simulink model "compare_filters"  (R2025a)
settings: Solver=VariableStepAuto  StartTime=0.0  StopTime=1.5  RelTol=1e-3
values from neighbouring files (symbols this model uses):
  phi_corr_LUT_param = Simulink.Parameter(phi_corr_LUT)    [lut_script.m]
undefined symbols (not defined in the file or in its folder): closed_loop, D_duty_cycle, D_m, DiscIntNeverNeededParam, hall_errors, I_duty_cycle, J_t, L_ss, lambda_m, P, P_duty_cycle, r_s, R_vs, T_m, theta_v, use_LUT, V_bus
libraries: spsMosfetLib x18, spsSeriesRLCBranchLib x12, spsVoltageMeasurementLib x9, spsControlledCurrentSourceLib x9, slpidlib x6, eeGeneralControl x3, simulink x3, embmathops x3, spsControlledVoltageSourceLib x3, spsPWMGeneratorDCDCLib x3, spsDCVoltageSourceLib x3, sps_lib x3
(part 2 of 3)

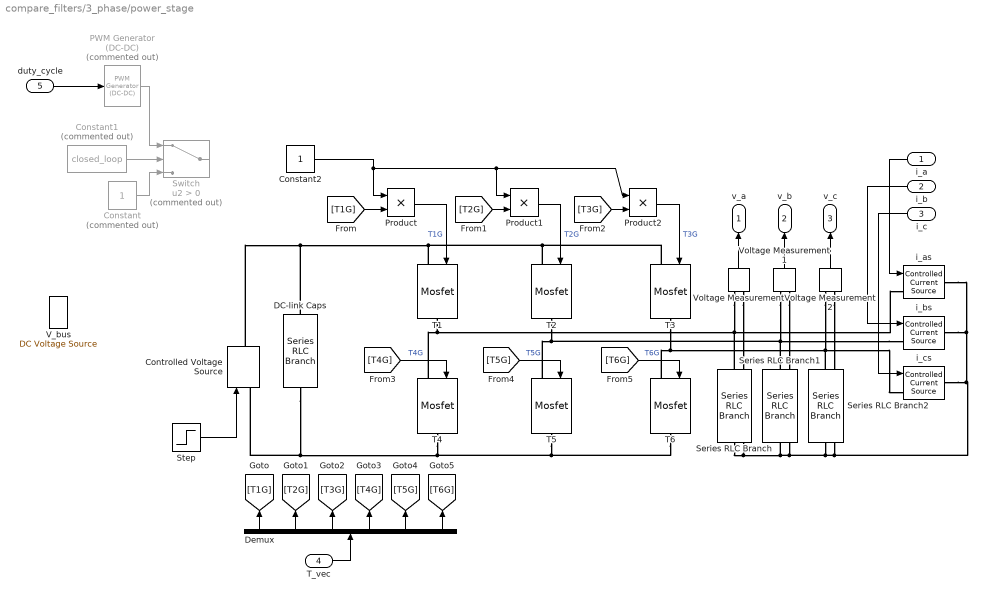
== system compare_filters/3_phase/power_stage ==
  i_a : Inport
  i_b : Inport  Port=2
  i_c : Inport  Port=3
  T_vec : Inport  Port=4
  duty_cycle : Inport  Port=5
  Constant : Constant  Commented=on
  Constant1 : Constant  Commented=on  Value=closed_loop
  Constant2 : Constant
  Controlled Voltage Source : spsControlledVoltageSourceLib/Controlled Voltage Source  Initialize=on  Source_Type=DC  Amplitude=20  Phase=0  Frequency=0  Measurements=None
  DC-link Caps : spsSeriesRLCBranchLib/Series RLC Branch  LConnTagsString=__new0  RConnTagsString=__new0  BranchType=RC  Resistance=1e-6  Inductance=0  SetiL0=off  InitialCurrent=0  Capacitance=100e-6  Setx0=off  InitialVoltage=0  Measurements=None
  Demux : Demux  Outputs=6
  PWM Generator (DC-DC) : spsPWMGeneratorDCDCLib/PWM Generator (DC-DC)  Commented=on  Fsw=f_SW_Hz  Ts=0
  Product : Product
  Product1 : Product
  Product2 : Product
  Series RLC Branch : spsSeriesRLCBranchLib/Series RLC Branch  LConnTagsString=__new0  RConnTagsString=__new0  BranchType=R  Resistance=R_vs  Inductance=0  SetiL0=off  InitialCurrent=0  Capacitance=inf  Setx0=off  InitialVoltage=0  Measurements=None
  Series RLC Branch1 : spsSeriesRLCBranchLib/Series RLC Branch  LConnTagsString=__new0  RConnTagsString=__new0  BranchType=R  Resistance=R_vs  Inductance=0  SetiL0=off  InitialCurrent=0  Capacitance=inf  Setx0=off  InitialVoltage=0  Measurements=None
  Series RLC Branch2 : spsSeriesRLCBranchLib/Series RLC Branch  LConnTagsString=__new0  RConnTagsString=__new0  BranchType=R  Resistance=R_vs  Inductance=0  SetiL0=off  InitialCurrent=0  Capacitance=inf  Setx0=off  InitialVoltage=0  Measurements=None
  Step : Step  Time=0.55  Before=20  After=35  SampleTime=0
  Switch : Switch  Commented=on  Criteria=u2 > Threshold  SaturateOnIntegerOverflow=off  InputSameDT=off
  T{1..6} (6 alike) : spsMosfetLib/Mosfet  Ron=R_dsON_Ohm  Lon=0  Rd=0.01  Vfd=0.7  IC=0  Rs=1e5  Cs=inf  Measurements=off
  V_bus : spsDCVoltageSourceLib/DC Voltage Source  Amplitude=V_bus  Measurements=None
  Voltage Measurement : spsVoltageMeasurementLib/Voltage Measurement  PhasorSimulation=off  OutputType=Complex  PSBequivalent=0
  Voltage Measurement1 : spsVoltageMeasurementLib/Voltage Measurement  PhasorSimulation=off  OutputType=Complex  PSBequivalent=0
  Voltage Measurement2 : spsVoltageMeasurementLib/Voltage Measurement  PhasorSimulation=off  OutputType=Complex  PSBequivalent=0
  i_as : spsControlledCurrentSourceLib/Controlled Current Source  Initialize=on  Source_Type=AC  Amplitude=0  Phase=0  Frequency=0  Measurements=None
  i_bs : spsControlledCurrentSourceLib/Controlled Current Source  Initialize=on  Source_Type=AC  Amplitude=0  Phase=0  Frequency=0  Measurements=None
  i_cs : spsControlledCurrentSourceLib/Controlled Current Source  Initialize=on  Source_Type=AC  Amplitude=0  Phase=0  Frequency=0  Measurements=None
  v_a : Outport
  v_b : Outport  Port=2
  v_c : Outport  Port=3
  wires:
  T_vec/1 -> Demux/1
  Product1/1 -> T2/1  "T2G"
  Constant2/1 -> Product/1, Product2/1, Product1/1
  Demux/6 -> [T6G]
  [T4G] -> T4/1  "T4G"
  [T5G] -> T5/1  "T5G"
  Demux/4 -> [T4G]
  Voltage Measurement/1 -> v_a/1
  [T2G] -> Product1/2
  Voltage Measurement1/1 -> v_b/1
  Voltage Measurement2/1 -> v_c/1
  i_a/1 -> i_as/1
  Demux/1 -> [T1G]
  Demux/5 -> [T5G]
  [T6G] -> T6/1  "T6G"
  i_c/1 -> i_cs/1
  Product/1 -> T1/1  "T1G"
  [T3G] -> Product2/2
  i_b/1 -> i_bs/1
  Product2/1 -> T3/1  "T3G"
  Demux/2 -> [T2G]
  Demux/3 -> [T3G]
  [T1G] -> Product/2
  duty_cycle/1 -> PWM Generator (DC-DC)/1
  Constant/1 -> Switch/3
  Constant1/1 -> Switch/2
  PWM Generator (DC-DC)/1 -> Switch/1
  Step/1 -> Controlled Voltage Source/1
  connections:
  i_bs/LConn1 -- Voltage Measurement1/LConn1 -- Series RLC Branch1/LConn1 -- T2/RConn1 -- T5/LConn1
  DC-link Caps/RConn1 -- Controlled Voltage Source/LConn1 -- T4/RConn1 -- T6/RConn1 -- T5/RConn1
  DC-link Caps/LConn1 -- Controlled Voltage Source/RConn1 -- T1/LConn1 -- T3/LConn1 -- T2/LConn1
  T4/LConn1 -- T1/RConn1 -- Voltage Measurement/LConn1 -- Series RLC Branch/LConn1 -- i_as/LConn1
  T3/RConn1 -- T6/LConn1 -- Voltage Measurement2/LConn1 -- Series RLC Branch2/LConn1 -- i_cs/LConn1
  Series RLC Branch/RConn1 -- Voltage Measurement/LConn2 -- i_bs/RConn1 -- i_as/RConn1 -- i_cs/RConn1 -- Voltage Measurement2/LConn2 -- Series RLC Branch2/RConn1 -- Voltage Measurement1/LConn2 -- Series RLC Branch1/RConn1

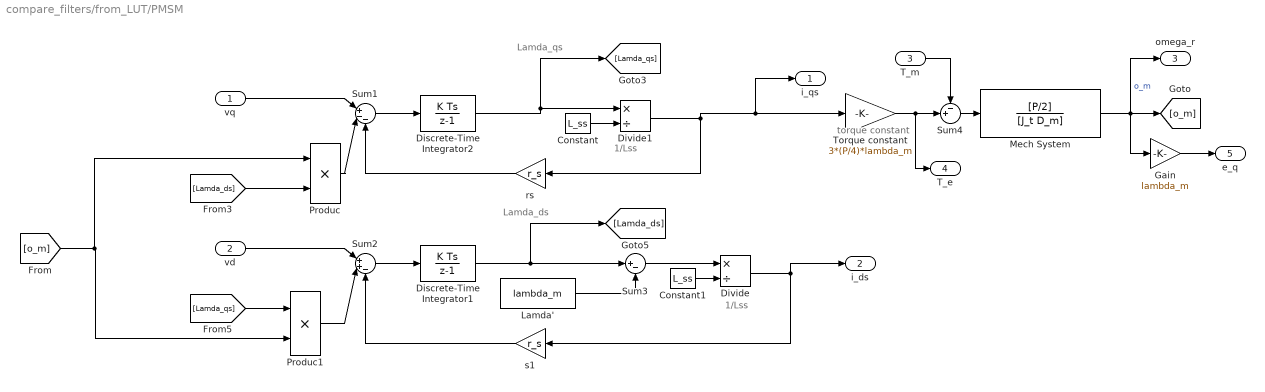
== system compare_filters/from_LUT/PMSM ==
  note: torque constant
  note: Lamda_ds
  note: Lamda_qs
  note: 1/Lss
  note: 1/Lss
  vq : Inport
  vd : Inport  Port=2
  T_m : Inport  Port=3
  Constant : Constant  Value=L_ss
  Constant1 : Constant  Value=L_ss
  Discrete-Time Integrator1 : DiscreteIntegrator  SampleTime=-1  ICPrevOutput=DiscIntNeverNeededParam  ICPrevScaledInput=DiscIntNeverNeededParam
  Discrete-Time Integrator2 : DiscreteIntegrator  SampleTime=-1  ICPrevOutput=DiscIntNeverNeededParam  ICPrevScaledInput=DiscIntNeverNeededParam
  Divide : Product  Inputs=*/
  Divide1 : Product  Inputs=*/
  Gain : Gain  Gain=lambda_m
  Lamda' : Constant  Value=lambda_m
  Mech System : TransferFcn  Numerator=[P/2]  Denominator=[J_t D_m]
  Produc : Product  RndMeth=Zero
  Produc1 : Product  RndMeth=Zero
  Sum1 : Sum  Inputs=|+--
  Sum2 : Sum  Inputs=|++-
  Sum3 : Sum  Inputs=|+-
  Sum4 : Sum  Inputs=-+|
  Torque constant : Gain  Gain=3*(P/4)*lambda_m
  rs : Gain  Gain=r_s
  s1 : Gain  Gain=r_s
  i_qs : Outport
  i_ds : Outport  Port=2
  omega_r : Outport  Port=3
  T_e : Outport  Port=4
  e_q : Outport  Port=5
  wires:
  vd/1 -> Sum2/1
  vq/1 -> Sum1/1
  [Lamda_qs] -> Produc1/1
  [Lamda_ds] -> Produc/2
  [o_m] -> Produc1/2, Produc/1
  Lamda'/1 -> Sum3/2
  Sum3/1 -> Divide/1
  s1/1 -> Sum2/3
  Discrete-Time Integrator1/1 -> [Lamda_ds], Sum3/1
  Sum2/1 -> Discrete-Time Integrator1/1
  Produc1/1 -> Sum2/2
  Divide1/1 -> i_qs/1, Torque constant/1, rs/1
  rs/1 -> Sum1/3
  Discrete-Time Integrator2/1 -> [Lamda_qs], Divide1/1
  Sum1/1 -> Discrete-Time Integrator2/1
  Produc/1 -> Sum1/2
  Torque constant/1 -> Sum4/2, T_e/1
  Divide/1 -> i_ds/1, s1/1
  T_m/1 -> Sum4/1
  Sum4/1 -> Mech System/1
  Constant/1 -> Divide1/2
  Constant1/1 -> Divide/2
  Mech System/1 -> Gain/1, omega_r/1, [o_m]  "o_m"
  Gain/1 -> e_q/1

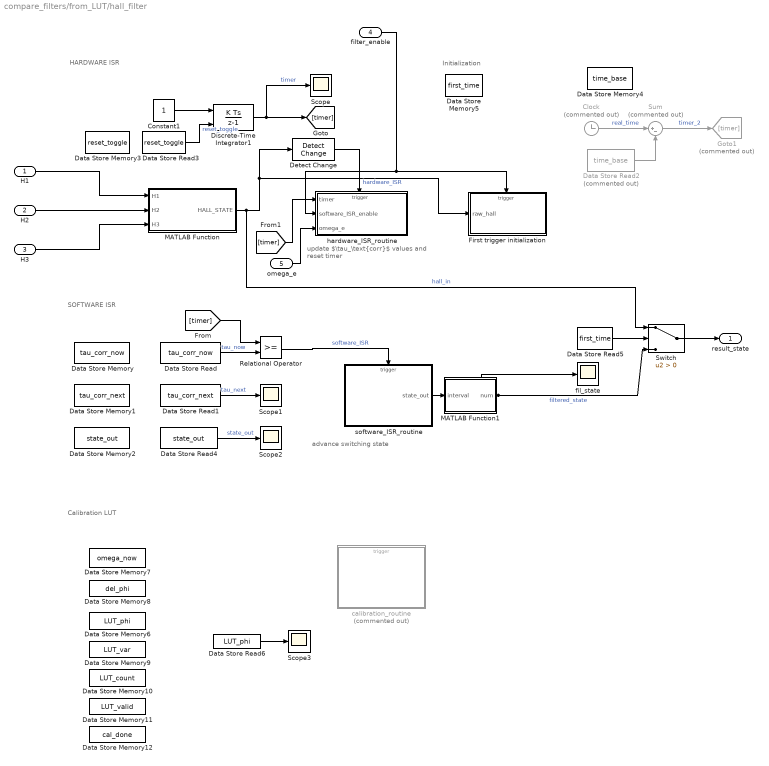
== system compare_filters/from_LUT/hall_filter ==
  note: Calibration LUT
  note: Initialization
  note: SOFTWARE ISR
  note: HARDWARE ISR
  note: update $\tau_\text{corr}$ values and reset timer
  note: advance switching state
  H1 : Inport
  H2 : Inport  Port=2
  H3 : Inport  Port=3
  filter_enable : Inport  Port=4
  omega_e : Inport  Port=5
  Clock : Clock  Commented=on
  Constant1 : Constant
  Data Store Memory : DataStoreMemory  DataStoreName=tau_corr_now  WriteAfterWriteMsg=warning  InitialValue=-1  ShowAdditionalParam=off
  Data Store Memory1 : DataStoreMemory  DataStoreName=tau_corr_next  WriteAfterWriteMsg=warning  InitialValue=-1  ShowAdditionalParam=off
  Data Store Memory10 : DataStoreMemory  DataStoreName=LUT_count  WriteAfterWriteMsg=warning  InitialValue=[0 0 0 0 0 0]  ShowAdditionalParam=off
  Data Store Memory11 : DataStoreMemory  DataStoreName=LUT_valid  WriteAfterWriteMsg=warning  InitialValue=[0 0 0 0 0 0]  ShowAdditionalParam=off
  Data Store Memory12 : DataStoreMemory  DataStoreName=cal_done  WriteAfterWriteMsg=warning  ShowAdditionalParam=off  OutDataTypeStr=boolean
  Data Store Memory2 : DataStoreMemory  DataStoreName=state_out  WriteAfterWriteMsg=warning  InitialValue=2  ShowAdditionalParam=off
  Data Store Memory3 : DataStoreMemory  DataStoreName=reset_toggle  WriteAfterWriteMsg=warning  ShowAdditionalParam=off
  Data Store Memory4 : DataStoreMemory  DataStoreName=time_base  WriteAfterWriteMsg=warning  ShowAdditionalParam=off
  Data Store Memory5 : DataStoreMemory  DataStoreName=first_time  WriteAfterWriteMsg=warning  InitialValue=1  ShowAdditionalParam=off
  Data Store Memory6 : DataStoreMemory  DataStoreName=LUT_phi  WriteAfterWriteMsg=warning  InitialValue=[0 0 0 0 0 0]  ShowAdditionalParam=off
  Data Store Memory7 : DataStoreMemory  DataStoreName=omega_now  WriteAfterWriteMsg=warning  ShowAdditionalParam=off
  Data Store Memory8 : DataStoreMemory  DataStoreName=del_phi  WriteAfterWriteMsg=warning  ShowAdditionalParam=off
  Data Store Memory9 : DataStoreMemory  DataStoreName=LUT_var  WriteAfterWriteMsg=warning  InitialValue=[0 0 0 0 0 0]  ShowAdditionalParam=off
  Data Store Read : DataStoreRead  DataStoreName=tau_corr_now  IndexOptions=Index vector (dialog)  Indices=1  OutputSizes=1
  Data Store Read1 : DataStoreRead  DataStoreName=tau_corr_next  IndexOptions=Index vector (dialog)  Indices=1  OutputSizes=1
  Data Store Read2 : DataStoreRead  Commented=on  DataStoreName=time_base  IndexOptions=Index vector (dialog)  Indices=1  OutputSizes=1
  Data Store Read3 : DataStoreRead  DataStoreName=reset_toggle  IndexOptions=Index vector (dialog)  Indices=1  OutputSizes=1
  Data Store Read4 : DataStoreRead  DataStoreName=state_out  IndexOptions=Index vector (dialog)  Indices=1  OutputSizes=1
  Data Store Read5 : DataStoreRead  DataStoreName=first_time  IndexOptions=Index vector (dialog)  Indices=1  OutputSizes=1
  Data Store Read6 : DataStoreRead  DataStoreName=LUT_phi  IndexOptions=Index vector (dialog)  Indices=1  OutputSizes=1
  Detect Change : simulink/Logic and Bit Operations/Detect Change  vinit=0  OutDataTypeStr=boolean
  Discrete-Time Integrator1 : DiscreteIntegrator  ExternalReset=either  SampleTime=1/(1e6)  ICPrevOutput=DiscIntNeverNeededParam  ICPrevScaledInput=DiscIntNeverNeededParam
  First trigger initialization : Subsystem  TreatAsAtomicUnit=on
  Goto1 : Goto  Commented=on  GotoTag=timer
  MATLAB Function : MATLAB Function  TreatAsAtomicUnit=on
  MATLAB Function1 : MATLAB Function  TreatAsAtomicUnit=on
  Relational Operator : RelationalOperator  OutDataTypeStr=boolean  RndMeth=Simplest  InputSameDT=off
  Scope{,1..3} (4 alike) : Scope
      Scope settings: ActiveDisplayYMinimum=-6.25  ActiveDisplayYMaximum=56.25
      Scope1 settings: ActiveDisplayYMinimum=7.96701  ActiveDisplayYMaximum=8.03137
      Scope2 settings: ActiveDisplayYMinimum=7.96701  ActiveDisplayYMaximum=8.03137
      Scope3 settings: ActiveDisplayYMinimum=0.99241576103971962  ActiveDisplayYMaximum=1.0799572702760518  DataLoggingVariableName=ScopeData2
  Sum : Sum  Commented=on  Inputs=|+-
  Switch : Switch  Criteria=u2 > Threshold  SaturateOnIntegerOverflow=off  InputSameDT=off
  calibration_routine : Subsystem  Priority=11  Commented=on  TreatAsAtomicUnit=on
  fil_state : Scope
      settings: ActiveDisplayYMinimum=-0.75  ActiveDisplayYMaximum=6.75  DataLoggingVariableName=ScopeData3
  hardware_ISR_routine : Subsystem  Priority=1
  software_ISR_routine : Subsystem  Priority=10  TreatAsAtomicUnit=on
  result_state : Outport
  wires:
  Discrete-Time Integrator1/1 -> [timer], Scope/1  "timer"
  Relational Operator/1 -> software_ISR_routine/Trigger  "software_ISR"
  Constant1/1 -> Discrete-Time Integrator1/1
  [timer] -> Relational Operator/1
  software_ISR_routine/1(state_out) -> MATLAB Function1/1(interval)
  MATLAB Function/1(HALL_STATE) -> Switch/1, Detect Change/1, First trigger initialization/1(raw_hall)  "hall_in"
  Data Store Read3/1 -> Discrete-Time Integrator1/2  "reset_toggle"
  Data Store Read1/1 -> Scope1/1  "tau_next"
  Data Store Read/1 -> Relational Operator/2  "tau_now"
  H3/1 -> MATLAB Function/3(H3)
  H2/1 -> MATLAB Function/2(H2)
  H1/1 -> MATLAB Function/1(H1)
  MATLAB Function1/1(num) -> fil_state/1, Switch/3  "filtered_state"
  Detect Change/1 -> hardware_ISR_routine/Trigger  "hardware_ISR"
  Data Store Read4/1 -> Scope2/1  "state_out"
  filter_enable/1 -> First trigger initialization/Trigger, hardware_ISR_routine/2(software_ISR_enable)
  Clock/1 -> Sum/1  "real_time"
  [timer] -> hardware_ISR_routine/1(timer)
  Data Store Read2/1 -> Sum/2
  Sum/1 -> Goto1/1  "timer_2"
  Data Store Read5/1 -> Switch/2
  Switch/1 -> result_state/1
  Data Store Read6/1 -> Scope3/1
  omega_e/1 -> hardware_ISR_routine/3(omega_e)

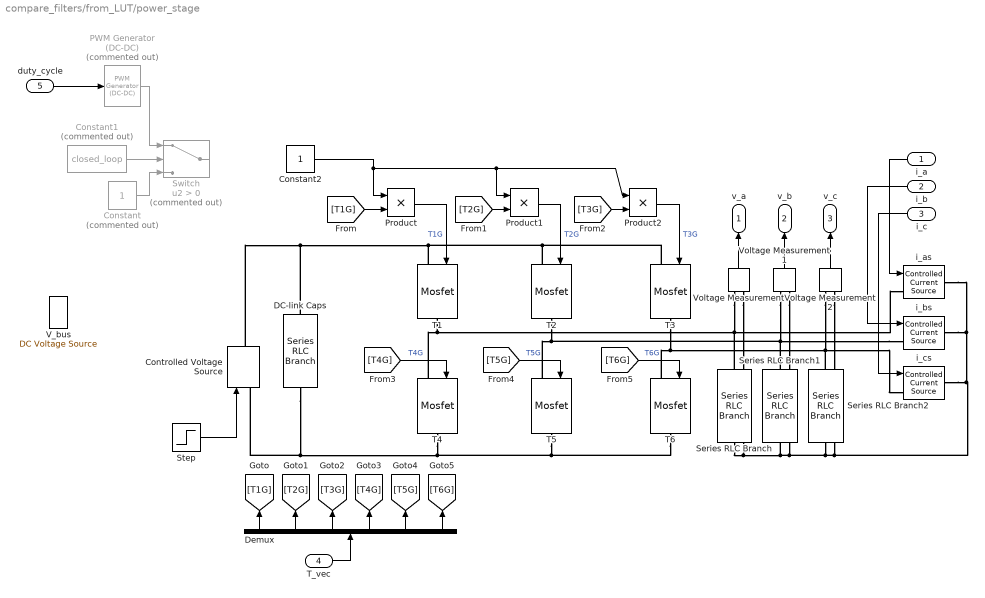
== system compare_filters/from_LUT/power_stage ==
  i_a : Inport
  i_b : Inport  Port=2
  i_c : Inport  Port=3
  T_vec : Inport  Port=4
  duty_cycle : Inport  Port=5
  Constant : Constant  Commented=on
  Constant1 : Constant  Commented=on  Value=closed_loop
  Constant2 : Constant
  Controlled Voltage Source : spsControlledVoltageSourceLib/Controlled Voltage Source  Initialize=on  Source_Type=DC  Amplitude=20  Phase=0  Frequency=0  Measurements=None
  DC-link Caps : spsSeriesRLCBranchLib/Series RLC Branch  LConnTagsString=__new0  RConnTagsString=__new0  BranchType=RC  Resistance=1e-6  Inductance=0  SetiL0=off  InitialCurrent=0  Capacitance=100e-6  Setx0=off  InitialVoltage=0  Measurements=None
  Demux : Demux  Outputs=6
  PWM Generator (DC-DC) : spsPWMGeneratorDCDCLib/PWM Generator (DC-DC)  Commented=on  Fsw=f_SW_Hz  Ts=0
  Product : Product
  Product1 : Product
  Product2 : Product
  Series RLC Branch : spsSeriesRLCBranchLib/Series RLC Branch  LConnTagsString=__new0  RConnTagsString=__new0  BranchType=R  Resistance=R_vs  Inductance=0  SetiL0=off  InitialCurrent=0  Capacitance=inf  Setx0=off  InitialVoltage=0  Measurements=None
  Series RLC Branch1 : spsSeriesRLCBranchLib/Series RLC Branch  LConnTagsString=__new0  RConnTagsString=__new0  BranchType=R  Resistance=R_vs  Inductance=0  SetiL0=off  InitialCurrent=0  Capacitance=inf  Setx0=off  InitialVoltage=0  Measurements=None
  Series RLC Branch2 : spsSeriesRLCBranchLib/Series RLC Branch  LConnTagsString=__new0  RConnTagsString=__new0  BranchType=R  Resistance=R_vs  Inductance=0  SetiL0=off  InitialCurrent=0  Capacitance=inf  Setx0=off  InitialVoltage=0  Measurements=None
  Step : Step  Time=0.55  Before=20  After=35  SampleTime=0
  Switch : Switch  Commented=on  Criteria=u2 > Threshold  SaturateOnIntegerOverflow=off  InputSameDT=off
  T{1..6} (6 alike) : spsMosfetLib/Mosfet  Ron=R_dsON_Ohm  Lon=0  Rd=0.01  Vfd=0.7  IC=0  Rs=1e5  Cs=inf  Measurements=off
  V_bus : spsDCVoltageSourceLib/DC Voltage Source  Amplitude=V_bus  Measurements=None
  Voltage Measurement : spsVoltageMeasurementLib/Voltage Measurement  PhasorSimulation=off  OutputType=Complex  PSBequivalent=0
  Voltage Measurement1 : spsVoltageMeasurementLib/Voltage Measurement  PhasorSimulation=off  OutputType=Complex  PSBequivalent=0
  Voltage Measurement2 : spsVoltageMeasurementLib/Voltage Measurement  PhasorSimulation=off  OutputType=Complex  PSBequivalent=0
  i_as : spsControlledCurrentSourceLib/Controlled Current Source  Initialize=on  Source_Type=AC  Amplitude=0  Phase=0  Frequency=0  Measurements=None
  i_bs : spsControlledCurrentSourceLib/Controlled Current Source  Initialize=on  Source_Type=AC  Amplitude=0  Phase=0  Frequency=0  Measurements=None
  i_cs : spsControlledCurrentSourceLib/Controlled Current Source  Initialize=on  Source_Type=AC  Amplitude=0  Phase=0  Frequency=0  Measurements=None
  v_a : Outport
  v_b : Outport  Port=2
  v_c : Outport  Port=3
  wires:
  T_vec/1 -> Demux/1
  Product1/1 -> T2/1  "T2G"
  Constant2/1 -> Product/1, Product2/1, Product1/1
  Demux/6 -> [T6G]
  [T4G] -> T4/1  "T4G"
  [T5G] -> T5/1  "T5G"
  Demux/4 -> [T4G]
  Voltage Measurement/1 -> v_a/1
  [T2G] -> Product1/2
  Voltage Measurement1/1 -> v_b/1
  Voltage Measurement2/1 -> v_c/1
  i_a/1 -> i_as/1
  Demux/1 -> [T1G]
  Demux/5 -> [T5G]
  [T6G] -> T6/1  "T6G"
  i_c/1 -> i_cs/1
  Product/1 -> T1/1  "T1G"
  [T3G] -> Product2/2
  i_b/1 -> i_bs/1
  Product2/1 -> T3/1  "T3G"
  Demux/2 -> [T2G]
  Demux/3 -> [T3G]
  [T1G] -> Product/2
  duty_cycle/1 -> PWM Generator (DC-DC)/1
  Constant/1 -> Switch/3
  Constant1/1 -> Switch/2
  PWM Generator (DC-DC)/1 -> Switch/1
  Step/1 -> Controlled Voltage Source/1
  connections:
  i_bs/LConn1 -- Voltage Measurement1/LConn1 -- Series RLC Branch1/LConn1 -- T2/RConn1 -- T5/LConn1
  DC-link Caps/RConn1 -- Controlled Voltage Source/LConn1 -- T4/RConn1 -- T6/RConn1 -- T5/RConn1
  DC-link Caps/LConn1 -- Controlled Voltage Source/RConn1 -- T1/LConn1 -- T3/LConn1 -- T2/LConn1
  T4/LConn1 -- T1/RConn1 -- Voltage Measurement/LConn1 -- Series RLC Branch/LConn1 -- i_as/LConn1
  T3/RConn1 -- T6/LConn1 -- Voltage Measurement2/LConn1 -- Series RLC Branch2/LConn1 -- i_cs/LConn1
  Series RLC Branch/RConn1 -- Voltage Measurement/LConn2 -- i_bs/RConn1 -- i_as/RConn1 -- i_cs/RConn1 -- Voltage Measurement2/LConn2 -- Series RLC Branch2/RConn1 -- Voltage Measurement1/LConn2 -- Series RLC Branch1/RConn1

== system compare_filters/no_LUT/PMSM ==
  note: torque constant
  note: Lamda_ds
  note: Lamda_qs
  note: 1/Lss
  note: 1/Lss
  vq : Inport
  vd : Inport  Port=2
  T_m : Inport  Port=3
  Constant : Constant  Value=L_ss
  Constant1 : Constant  Value=L_ss
  Discrete-Time Integrator1 : DiscreteIntegrator  SampleTime=-1  ICPrevOutput=DiscIntNeverNeededParam  ICPrevScaledInput=DiscIntNeverNeededParam
  Discrete-Time Integrator2 : DiscreteIntegrator  SampleTime=-1  ICPrevOutput=DiscIntNeverNeededParam  ICPrevScaledInput=DiscIntNeverNeededParam
  Divide : Product  Inputs=*/
  Divide1 : Product  Inputs=*/
  Gain : Gain  Gain=lambda_m
  Lamda' : Constant  Value=lambda_m
  Mech System : TransferFcn  Numerator=[P/2]  Denominator=[J_t D_m]
  Produc : Product  RndMeth=Zero
  Produc1 : Product  RndMeth=Zero
  Sum1 : Sum  Inputs=|+--
  Sum2 : Sum  Inputs=|++-
  Sum3 : Sum  Inputs=|+-
  Sum4 : Sum  Inputs=-+|
  Torque constant : Gain  Gain=3*(P/4)*lambda_m
  rs : Gain  Gain=r_s
  s1 : Gain  Gain=r_s
  i_qs : Outport
  i_ds : Outport  Port=2
  omega_r : Outport  Port=3
  T_e : Outport  Port=4
  e_q : Outport  Port=5
  wires:
  vd/1 -> Sum2/1
  vq/1 -> Sum1/1
  [Lamda_qs] -> Produc1/1
  [Lamda_ds] -> Produc/2
  [o_m] -> Produc1/2, Produc/1
  Lamda'/1 -> Sum3/2
  Sum3/1 -> Divide/1
  s1/1 -> Sum2/3
  Discrete-Time Integrator1/1 -> [Lamda_ds], Sum3/1
  Sum2/1 -> Discrete-Time Integrator1/1
  Produc1/1 -> Sum2/2
  Divide1/1 -> i_qs/1, Torque constant/1, rs/1
  rs/1 -> Sum1/3
  Discrete-Time Integrator2/1 -> [Lamda_qs], Divide1/1
  Sum1/1 -> Discrete-Time Integrator2/1
  Produc/1 -> Sum1/2
  Torque constant/1 -> Sum4/2, T_e/1
  Divide/1 -> i_ds/1, s1/1
  T_m/1 -> Sum4/1
  Sum4/1 -> Mech System/1
  Constant/1 -> Divide1/2
  Constant1/1 -> Divide/2
  Mech System/1 -> Gain/1, omega_r/1, [o_m]  "o_m"
  Gain/1 -> e_q/1

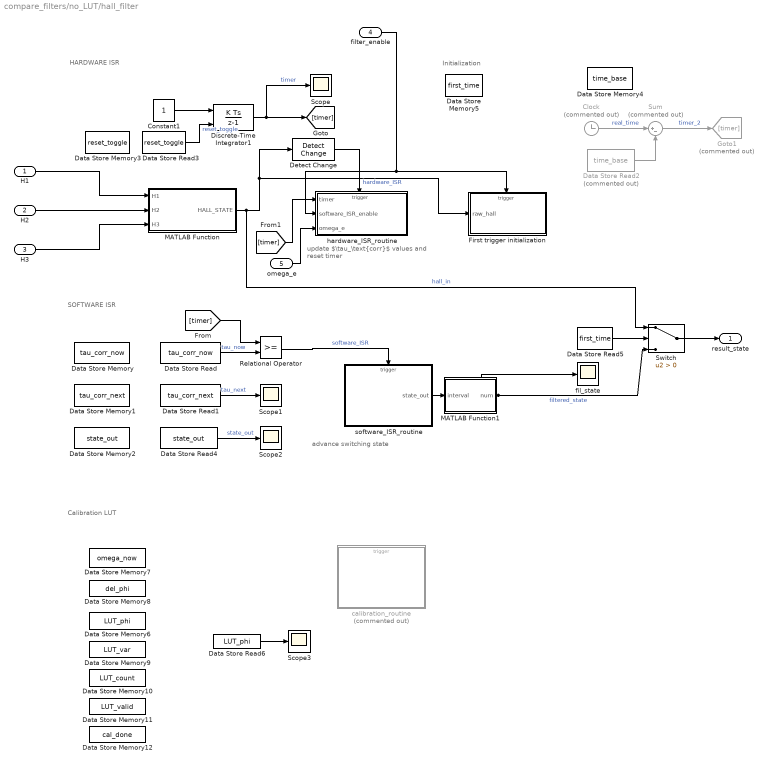
== system compare_filters/no_LUT/hall_filter ==
  note: Calibration LUT
  note: Initialization
  note: SOFTWARE ISR
  note: HARDWARE ISR
  note: update $\tau_\text{corr}$ values and reset timer
  note: advance switching state
  H1 : Inport
  H2 : Inport  Port=2
  H3 : Inport  Port=3
  filter_enable : Inport  Port=4
  omega_e : Inport  Port=5
  Clock : Clock  Commented=on
  Constant1 : Constant
  Data Store Memory : DataStoreMemory  DataStoreName=tau_corr_now  WriteAfterWriteMsg=warning  InitialValue=-1  ShowAdditionalParam=off
  Data Store Memory1 : DataStoreMemory  DataStoreName=tau_corr_next  WriteAfterWriteMsg=warning  InitialValue=-1  ShowAdditionalParam=off
  Data Store Memory10 : DataStoreMemory  DataStoreName=LUT_count  WriteAfterWriteMsg=warning  InitialValue=[0 0 0 0 0 0]  ShowAdditionalParam=off
  Data Store Memory11 : DataStoreMemory  DataStoreName=LUT_valid  WriteAfterWriteMsg=warning  InitialValue=[0 0 0 0 0 0]  ShowAdditionalParam=off
  Data Store Memory12 : DataStoreMemory  DataStoreName=cal_done  WriteAfterWriteMsg=warning  ShowAdditionalParam=off  OutDataTypeStr=boolean
  Data Store Memory2 : DataStoreMemory  DataStoreName=state_out  WriteAfterWriteMsg=warning  InitialValue=2  ShowAdditionalParam=off
  Data Store Memory3 : DataStoreMemory  DataStoreName=reset_toggle  WriteAfterWriteMsg=warning  ShowAdditionalParam=off
  Data Store Memory4 : DataStoreMemory  DataStoreName=time_base  WriteAfterWriteMsg=warning  ShowAdditionalParam=off
  Data Store Memory5 : DataStoreMemory  DataStoreName=first_time  WriteAfterWriteMsg=warning  InitialValue=1  ShowAdditionalParam=off
  Data Store Memory6 : DataStoreMemory  DataStoreName=LUT_phi  WriteAfterWriteMsg=warning  InitialValue=[0 0 0 0 0 0]  ShowAdditionalParam=off
  Data Store Memory7 : DataStoreMemory  DataStoreName=omega_now  WriteAfterWriteMsg=warning  ShowAdditionalParam=off
  Data Store Memory8 : DataStoreMemory  DataStoreName=del_phi  WriteAfterWriteMsg=warning  ShowAdditionalParam=off
  Data Store Memory9 : DataStoreMemory  DataStoreName=LUT_var  WriteAfterWriteMsg=warning  InitialValue=[0 0 0 0 0 0]  ShowAdditionalParam=off
  Data Store Read : DataStoreRead  DataStoreName=tau_corr_now  IndexOptions=Index vector (dialog)  Indices=1  OutputSizes=1
  Data Store Read1 : DataStoreRead  DataStoreName=tau_corr_next  IndexOptions=Index vector (dialog)  Indices=1  OutputSizes=1
  Data Store Read2 : DataStoreRead  Commented=on  DataStoreName=time_base  IndexOptions=Index vector (dialog)  Indices=1  OutputSizes=1
  Data Store Read3 : DataStoreRead  DataStoreName=reset_toggle  IndexOptions=Index vector (dialog)  Indices=1  OutputSizes=1
  Data Store Read4 : DataStoreRead  DataStoreName=state_out  IndexOptions=Index vector (dialog)  Indices=1  OutputSizes=1
  Data Store Read5 : DataStoreRead  DataStoreName=first_time  IndexOptions=Index vector (dialog)  Indices=1  OutputSizes=1
  Data Store Read6 : DataStoreRead  DataStoreName=LUT_phi  IndexOptions=Index vector (dialog)  Indices=1  OutputSizes=1
  Detect Change : simulink/Logic and Bit Operations/Detect Change  vinit=0  OutDataTypeStr=boolean
  Discrete-Time Integrator1 : DiscreteIntegrator  ExternalReset=either  SampleTime=1/(1e6)  ICPrevOutput=DiscIntNeverNeededParam  ICPrevScaledInput=DiscIntNeverNeededParam
  First trigger initialization : Subsystem  TreatAsAtomicUnit=on
  Goto1 : Goto  Commented=on  GotoTag=timer
  MATLAB Function : MATLAB Function  TreatAsAtomicUnit=on
  MATLAB Function1 : MATLAB Function  TreatAsAtomicUnit=on
  Relational Operator : RelationalOperator  OutDataTypeStr=boolean  RndMeth=Simplest  InputSameDT=off
  Scope{,1..3} (4 alike) : Scope
      Scope settings: ActiveDisplayYMinimum=-6.25  ActiveDisplayYMaximum=56.25
      Scope1 settings: ActiveDisplayYMinimum=7.96701  ActiveDisplayYMaximum=8.03137
      Scope2 settings: ActiveDisplayYMinimum=7.96701  ActiveDisplayYMaximum=8.03137
      Scope3 settings: ActiveDisplayYMinimum=0.99241576103971962  ActiveDisplayYMaximum=1.0799572702760518  DataLoggingVariableName=ScopeData2
  Sum : Sum  Commented=on  Inputs=|+-
  Switch : Switch  Criteria=u2 > Threshold  SaturateOnIntegerOverflow=off  InputSameDT=off
  calibration_routine : Subsystem  Priority=11  Commented=on  TreatAsAtomicUnit=on
  fil_state : Scope
      settings: ActiveDisplayYMinimum=-0.75  ActiveDisplayYMaximum=6.75  DataLoggingVariableName=ScopeData3
  hardware_ISR_routine : Subsystem  Priority=1
  software_ISR_routine : Subsystem  Priority=10  TreatAsAtomicUnit=on
  result_state : Outport
  wires:
  Discrete-Time Integrator1/1 -> [timer], Scope/1  "timer"
  Relational Operator/1 -> software_ISR_routine/Trigger  "software_ISR"
  Constant1/1 -> Discrete-Time Integrator1/1
  [timer] -> Relational Operator/1
  software_ISR_routine/1(state_out) -> MATLAB Function1/1(interval)
  MATLAB Function/1(HALL_STATE) -> Switch/1, Detect Change/1, First trigger initialization/1(raw_hall)  "hall_in"
  Data Store Read3/1 -> Discrete-Time Integrator1/2  "reset_toggle"
  Data Store Read1/1 -> Scope1/1  "tau_next"
  Data Store Read/1 -> Relational Operator/2  "tau_now"
  H3/1 -> MATLAB Function/3(H3)
  H2/1 -> MATLAB Function/2(H2)
  H1/1 -> MATLAB Function/1(H1)
  MATLAB Function1/1(num) -> fil_state/1, Switch/3  "filtered_state"
  Detect Change/1 -> hardware_ISR_routine/Trigger  "hardware_ISR"
  Data Store Read4/1 -> Scope2/1  "state_out"
  filter_enable/1 -> First trigger initialization/Trigger, hardware_ISR_routine/2(software_ISR_enable)
  Clock/1 -> Sum/1  "real_time"
  [timer] -> hardware_ISR_routine/1(timer)
  Data Store Read2/1 -> Sum/2
  Sum/1 -> Goto1/1  "timer_2"
  Data Store Read5/1 -> Switch/2
  Switch/1 -> result_state/1
  Data Store Read6/1 -> Scope3/1
  omega_e/1 -> hardware_ISR_routine/3(omega_e)

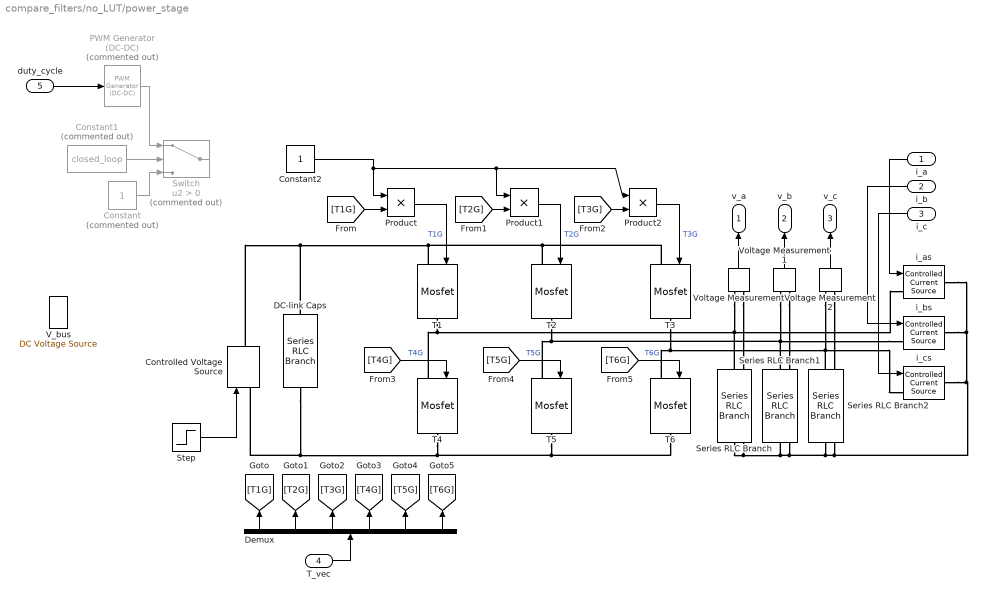
== system compare_filters/no_LUT/power_stage ==
  i_a : Inport
  i_b : Inport  Port=2
  i_c : Inport  Port=3
  T_vec : Inport  Port=4
  duty_cycle : Inport  Port=5
  Constant : Constant  Commented=on
  Constant1 : Constant  Commented=on  Value=closed_loop
  Constant2 : Constant
  Controlled Voltage Source : spsControlledVoltageSourceLib/Controlled Voltage Source  Initialize=on  Source_Type=DC  Amplitude=20  Phase=0  Frequency=0  Measurements=None
  DC-link Caps : spsSeriesRLCBranchLib/Series RLC Branch  LConnTagsString=__new0  RConnTagsString=__new0  BranchType=RC  Resistance=1e-6  Inductance=0  SetiL0=off  InitialCurrent=0  Capacitance=100e-6  Setx0=off  InitialVoltage=0  Measurements=None
  Demux : Demux  Outputs=6
  PWM Generator (DC-DC) : spsPWMGeneratorDCDCLib/PWM Generator (DC-DC)  Commented=on  Fsw=f_SW_Hz  Ts=0
  Product : Product
  Product1 : Product
  Product2 : Product
  Series RLC Branch : spsSeriesRLCBranchLib/Series RLC Branch  LConnTagsString=__new0  RConnTagsString=__new0  BranchType=R  Resistance=R_vs  Inductance=0  SetiL0=off  InitialCurrent=0  Capacitance=inf  Setx0=off  InitialVoltage=0  Measurements=None
  Series RLC Branch1 : spsSeriesRLCBranchLib/Series RLC Branch  LConnTagsString=__new0  RConnTagsString=__new0  BranchType=R  Resistance=R_vs  Inductance=0  SetiL0=off  InitialCurrent=0  Capacitance=inf  Setx0=off  InitialVoltage=0  Measurements=None
  Series RLC Branch2 : spsSeriesRLCBranchLib/Series RLC Branch  LConnTagsString=__new0  RConnTagsString=__new0  BranchType=R  Resistance=R_vs  Inductance=0  SetiL0=off  InitialCurrent=0  Capacitance=inf  Setx0=off  InitialVoltage=0  Measurements=None
  Step : Step  Time=0.55  Before=20  After=35  SampleTime=0
  Switch : Switch  Commented=on  Criteria=u2 > Threshold  SaturateOnIntegerOverflow=off  InputSameDT=off
  T{1..6} (6 alike) : spsMosfetLib/Mosfet  Ron=R_dsON_Ohm  Lon=0  Rd=0.01  Vfd=0.7  IC=0  Rs=1e5  Cs=inf  Measurements=off
  V_bus : spsDCVoltageSourceLib/DC Voltage Source  Amplitude=V_bus  Measurements=None
  Voltage Measurement : spsVoltageMeasurementLib/Voltage Measurement  PhasorSimulation=off  OutputType=Complex  PSBequivalent=0
  Voltage Measurement1 : spsVoltageMeasurementLib/Voltage Measurement  PhasorSimulation=off  OutputType=Complex  PSBequivalent=0
  Voltage Measurement2 : spsVoltageMeasurementLib/Voltage Measurement  PhasorSimulation=off  OutputType=Complex  PSBequivalent=0
  i_as : spsControlledCurrentSourceLib/Controlled Current Source  Initialize=on  Source_Type=AC  Amplitude=0  Phase=0  Frequency=0  Measurements=None
  i_bs : spsControlledCurrentSourceLib/Controlled Current Source  Initialize=on  Source_Type=AC  Amplitude=0  Phase=0  Frequency=0  Measurements=None
  i_cs : spsControlledCurrentSourceLib/Controlled Current Source  Initialize=on  Source_Type=AC  Amplitude=0  Phase=0  Frequency=0  Measurements=None
  v_a : Outport
  v_b : Outport  Port=2
  v_c : Outport  Port=3
  wires:
  T_vec/1 -> Demux/1
  Product1/1 -> T2/1  "T2G"
  Constant2/1 -> Product/1, Product2/1, Product1/1
  Demux/6 -> [T6G]
  [T4G] -> T4/1  "T4G"
  [T5G] -> T5/1  "T5G"
  Demux/4 -> [T4G]
  Voltage Measurement/1 -> v_a/1
  [T2G] -> Product1/2
  Voltage Measurement1/1 -> v_b/1
  Voltage Measurement2/1 -> v_c/1
  i_a/1 -> i_as/1
  Demux/1 -> [T1G]
  Demux/5 -> [T5G]
  [T6G] -> T6/1  "T6G"
  i_c/1 -> i_cs/1
  Product/1 -> T1/1  "T1G"
  [T3G] -> Product2/2
  i_b/1 -> i_bs/1
  Product2/1 -> T3/1  "T3G"
  Demux/2 -> [T2G]
  Demux/3 -> [T3G]
  [T1G] -> Product/2
  duty_cycle/1 -> PWM Generator (DC-DC)/1
  Constant/1 -> Switch/3
  Constant1/1 -> Switch/2
  PWM Generator (DC-DC)/1 -> Switch/1
  Step/1 -> Controlled Voltage Source/1
  connections:
  i_bs/LConn1 -- Voltage Measurement1/LConn1 -- Series RLC Branch1/LConn1 -- T2/RConn1 -- T5/LConn1
  DC-link Caps/RConn1 -- Controlled Voltage Source/LConn1 -- T4/RConn1 -- T6/RConn1 -- T5/RConn1
  DC-link Caps/LConn1 -- Controlled Voltage Source/RConn1 -- T1/LConn1 -- T3/LConn1 -- T2/LConn1
  T4/LConn1 -- T1/RConn1 -- Voltage Measurement/LConn1 -- Series RLC Branch/LConn1 -- i_as/LConn1
  T3/RConn1 -- T6/LConn1 -- Voltage Measurement2/LConn1 -- Series RLC Branch2/LConn1 -- i_cs/LConn1
  Series RLC Branch/RConn1 -- Voltage Measurement/LConn2 -- i_bs/RConn1 -- i_as/RConn1 -- i_cs/RConn1 -- Voltage Measurement2/LConn2 -- Series RLC Branch2/RConn1 -- Voltage Measurement1/LConn2 -- Series RLC Branch1/RConn1

== system compare_filters/3_phase/hall_filter/First trigger initialization ==
  note: no need to shift because the hall signal here is already late by 1
  raw_hall : Inport
  Trigger : TriggerPort  VariantControl=(inherit)  PortDimensions=1
  Constant : Constant  Value=0
  Data Store Write3 : DataStoreWrite  DataStoreName=state_out  IndexOptions=Index vector (dialog)  Indices=1  OutputSizes=1
  MATLAB Function : MATLAB Function  TreatAsAtomicUnit=on
  Sum : Sum  Inputs=|+-
  wires:
  raw_hall/1 -> MATLAB Function/1(num)
  MATLAB Function/1(interval) -> Sum/1
  Sum/1 -> Data Store Write3/1
  Constant/1 -> Sum/2

== system compare_filters/3_phase/hall_filter/calibration_routine ==
  note: $calculate ~\omega$
  note: $calculate ~\Delta\phi$
  note: $update ~LUT ~ table$
  function : TriggerPort  VariantControl=(inherit)
  Subsystem : Subsystem  Priority=11
  Subsystem1 : Subsystem  Priority=12
  Subsystem2 : Subsystem  Priority=13

== system compare_filters/3_phase/hall_filter/hardware_ISR_routine ==
  note: partially resolved edge case: when hardware ISR and software ISR coincide
  note: 2. toggle timer reset
  note: 3. calculate tau's
  note: 4. calculate and register tau values into queue
  note: 1. save current time
  timer : Inport
  software_ISR_enable : Inport  Port=2
  omega_e : Inport  Port=3
  Trigger : TriggerPort  VariantControl=(inherit)  PortDimensions=1
  Atomic Subsystem : Subsystem  Priority=5  TreatAsAtomicUnit=on
  Bias : Bias  Bias=1  SaturateOnIntegerOverflow=off
  Constant : Constant  Value=use_LUT
  Constant7 : Constant  Value=phi_corr_LUT_param
  Data Store Memory : DataStoreMemory  DataStoreName=t_now  WriteAfterWriteMsg=warning  ShowAdditionalParam=off
  Data Store Memory1 : DataStoreMemory  DataStoreName=tau_corr_out  WriteAfterWriteMsg=warning  ShowAdditionalParam=off
  Data Store Read : DataStoreRead  DataStoreName=t_now  IndexOptions=Index vector (dialog)  Indices=1  OutputSizes=1
  Data Store Read1 : DataStoreRead  DataStoreName=tau_corr_now  IndexOptions=Index vector (dialog)  Indices=1  OutputSizes=1
  Data Store Read2 : DataStoreRead  DataStoreName=tau_corr_next  IndexOptions=Index vector (dialog)  Indices=1  OutputSizes=1
  Data Store Read3 : DataStoreRead  DataStoreName=tau_corr_out  IndexOptions=Index vector (dialog)  Indices=1  OutputSizes=1
  Data Store Read5 : DataStoreRead  DataStoreName=state_out  IndexOptions=Index vector (dialog)  Indices=1  OutputSizes=1
  Data Store Read6 : DataStoreRead  DataStoreName=state_out  IndexOptions=Index vector (dialog)  Indices=1  OutputSizes=1
  Data Store Write : DataStoreWrite  DataStoreName=tau_corr_out  IndexOptions=Index vector (dialog)  Indices=1  OutputSizes=1
  Divide : Product  Inputs=*/
  MATLAB Function : MATLAB Function  Priority=4  TreatAsAtomicUnit=on
  MATLAB Function1 : MATLAB Function  TreatAsAtomicUnit=on
  Scope : Scope
      settings: ActiveDisplayYMinimum=-0.027793962383284257  ActiveDisplayYMaximum=0.030008936086375265  DataLoggingVariableName=ScopeData4
  Selector : Selector  InputPortWidth=6  IndexOptions=Index vector (port)  Indices=[1 3]  OutputSizes=1
  Selector1 : Selector  InputPortWidth=6  IndexOptions=Index vector (port)  Indices=[1 3]  OutputSizes=1
  Subsystem : Subsystem  Priority=2  Commented=on
  Subsystem1 : Subsystem  Priority=3
  Subsystem2 : Subsystem  Priority=1
  Subsystem3 : Subsystem  Priority=5  Commented=on
  Unit Delay : UnitDelay  SampleTime=-1  HasFrameUpgradeWarning=on
  wires:
  Data Store Read/1 -> MATLAB Function/1(timer), Subsystem1/1(In1)
  Data Store Read1/1 -> MATLAB Function/3(tau_now)  "tau_corr_now"
  timer/1 -> Subsystem2/1(timer)
  Subsystem1/1(tau_vec) -> MATLAB Function/2(tau_vec)
  MATLAB Function/1(tau_now_out) -> Atomic Subsystem/1(tau_now_write)  "tau_now_write"
  MATLAB Function/2(tau_next_out) -> Atomic Subsystem/2(tau_next_write)  "tau_next_write"
  software_ISR_enable/1 -> Atomic Subsystem/Enable
  MATLAB Function/3(update_now) -> Atomic Subsystem/3(update_now)
  MATLAB Function/4(update_next) -> Atomic Subsystem/4(update_next)
  MATLAB Function/5(tau_corr_out) -> Data Store Write/1
  Data Store Read3/1 -> Scope/1  "tau_corr_out"
  Data Store Read2/1 -> MATLAB Function/4(tau_next)
  Constant/1 -> MATLAB Function/6(use_LUT)
  Constant7/1 -> Selector1/1, Divide/1
  Divide/1 -> MATLAB Function1/1(tau_LUT_input), Selector/1, MATLAB Function/5(tau_LUT_input)
  omega_e/1 -> Divide/2
  Bias/1 -> Selector1/2, Selector/2
  Selector/1 -> ?  "tau_corr_LUT"
  Data Store Read5/1 -> MATLAB Function/7(state_out)
  Selector1/1 -> ?  "phi_corr_test"
  Data Store Read6/1 -> Bias/1
  MATLAB Function1/1(tau_corr_LUT_test) -> ?  "tau_corr_LUT_algo"

== system compare_filters/3_phase/hall_filter/software_ISR_routine ==
  note: turn off initialization flag
      | (only meaningful after initialization)
  note: advance switching state
  note: $\tau_\text{corr, next} -> \tau_\text{corr, now}$
  note: Update $\tau_\text{corr, next}$
  note: transfert state_out to output
  function : TriggerPort  VariantControl=(inherit)
  Subsystem : Subsystem  Priority=11
  Subsystem1 : Subsystem  Priority=12
  Subsystem2 : Subsystem  Priority=13
  Subsystem3 : Subsystem  Priority=14
  Subsystem4 : Subsystem  Priority=11
  state_out : Outport
  wires:
  Subsystem3/1(state_out) -> state_out/1

== system compare_filters/from_LUT/hall_filter/First trigger initialization ==
  note: no need to shift because the hall signal here is already late by 1
  raw_hall : Inport
  Trigger : TriggerPort  VariantControl=(inherit)  PortDimensions=1
  Constant : Constant  Value=0
  Data Store Write3 : DataStoreWrite  DataStoreName=state_out  IndexOptions=Index vector (dialog)  Indices=1  OutputSizes=1
  MATLAB Function : MATLAB Function  TreatAsAtomicUnit=on
  Sum : Sum  Inputs=|+-
  wires:
  raw_hall/1 -> MATLAB Function/1(num)
  MATLAB Function/1(interval) -> Sum/1
  Sum/1 -> Data Store Write3/1
  Constant/1 -> Sum/2

== system compare_filters/from_LUT/hall_filter/calibration_routine ==
  note: $calculate ~\omega$
  note: $calculate ~\Delta\phi$
  note: $update ~LUT ~ table$
  function : TriggerPort  VariantControl=(inherit)
  Subsystem : Subsystem  Priority=11
  Subsystem1 : Subsystem  Priority=12
  Subsystem2 : Subsystem  Priority=13

== system compare_filters/from_LUT/hall_filter/hardware_ISR_routine ==
  note: partially resolved edge case: when hardware ISR and software ISR coincide
  note: 2. toggle timer reset
  note: 3. calculate tau's
  note: 4. calculate and register tau values into queue
  note: 1. save current time
  timer : Inport
  software_ISR_enable : Inport  Port=2
  omega_e : Inport  Port=3
  Trigger : TriggerPort  VariantControl=(inherit)  PortDimensions=1
  Atomic Subsystem : Subsystem  Priority=5  TreatAsAtomicUnit=on
  Bias : Bias  Bias=1  SaturateOnIntegerOverflow=off
  Constant : Constant  Value=use_LUT
  Constant7 : Constant  Value=phi_corr_LUT_param
  Data Store Memory : DataStoreMemory  DataStoreName=t_now  WriteAfterWriteMsg=warning  ShowAdditionalParam=off
  Data Store Memory1 : DataStoreMemory  DataStoreName=tau_corr_out  WriteAfterWriteMsg=warning  ShowAdditionalParam=off
  Data Store Read : DataStoreRead  DataStoreName=t_now  IndexOptions=Index vector (dialog)  Indices=1  OutputSizes=1
  Data Store Read1 : DataStoreRead  DataStoreName=tau_corr_now  IndexOptions=Index vector (dialog)  Indices=1  OutputSizes=1
  Data Store Read2 : DataStoreRead  DataStoreName=tau_corr_next  IndexOptions=Index vector (dialog)  Indices=1  OutputSizes=1
  Data Store Read3 : DataStoreRead  DataStoreName=tau_corr_out  IndexOptions=Index vector (dialog)  Indices=1  OutputSizes=1
  Data Store Read5 : DataStoreRead  DataStoreName=state_out  IndexOptions=Index vector (dialog)  Indices=1  OutputSizes=1
  Data Store Read6 : DataStoreRead  DataStoreName=state_out  IndexOptions=Index vector (dialog)  Indices=1  OutputSizes=1
  Data Store Write : DataStoreWrite  DataStoreName=tau_corr_out  IndexOptions=Index vector (dialog)  Indices=1  OutputSizes=1
  Divide : Product  Inputs=*/
  MATLAB Function : MATLAB Function  Priority=4  TreatAsAtomicUnit=on
  MATLAB Function1 : MATLAB Function  TreatAsAtomicUnit=on
  Scope : Scope
      settings: ActiveDisplayYMinimum=-0.027793962383284257  ActiveDisplayYMaximum=0.030008936086375265  DataLoggingVariableName=ScopeData4
  Selector : Selector  InputPortWidth=6  IndexOptions=Index vector (port)  Indices=[1 3]  OutputSizes=1
  Selector1 : Selector  InputPortWidth=6  IndexOptions=Index vector (port)  Indices=[1 3]  OutputSizes=1
  Subsystem : Subsystem  Priority=2  Commented=on
  Subsystem1 : Subsystem  Priority=3
  Subsystem2 : Subsystem  Priority=1
  Subsystem3 : Subsystem  Priority=5  Commented=on
  Unit Delay : UnitDelay  SampleTime=-1  HasFrameUpgradeWarning=on
  wires:
  Data Store Read/1 -> MATLAB Function/1(timer), Subsystem1/1(In1)
  Data Store Read1/1 -> MATLAB Function/3(tau_now)  "tau_corr_now"
  timer/1 -> Subsystem2/1(timer)
  Subsystem1/1(tau_vec) -> MATLAB Function/2(tau_vec)
  MATLAB Function/1(tau_now_out) -> Atomic Subsystem/1(tau_now_write)  "tau_now_write"
  MATLAB Function/2(tau_next_out) -> Atomic Subsystem/2(tau_next_write)  "tau_next_write"
  software_ISR_enable/1 -> Atomic Subsystem/Enable
  MATLAB Function/3(update_now) -> Atomic Subsystem/3(update_now)
  MATLAB Function/4(update_next) -> Atomic Subsystem/4(update_next)
  MATLAB Function/5(tau_corr_out) -> Data Store Write/1
  Data Store Read3/1 -> Scope/1  "tau_corr_out"
  Data Store Read2/1 -> MATLAB Function/4(tau_next)
  Constant/1 -> MATLAB Function/6(use_LUT)
  Constant7/1 -> Selector1/1, Divide/1
  Divide/1 -> MATLAB Function1/1(tau_LUT_input), Selector/1, MATLAB Function/5(tau_LUT_input)
  omega_e/1 -> Divide/2
  Bias/1 -> Selector1/2, Selector/2
  Selector/1 -> ?  "tau_corr_LUT"
  Data Store Read5/1 -> MATLAB Function/7(state_out)
  Selector1/1 -> ?  "phi_corr_test"
  Data Store Read6/1 -> Bias/1
  MATLAB Function1/1(tau_corr_LUT_test) -> ?  "tau_corr_LUT_algo"

== system compare_filters/from_LUT/hall_filter/software_ISR_routine ==
  note: turn off initialization flag
      | (only meaningful after initialization)
  note: advance switching state
  note: $\tau_\text{corr, next} -> \tau_\text{corr, now}$
  note: Update $\tau_\text{corr, next}$
  note: transfert state_out to output
  function : TriggerPort  VariantControl=(inherit)
  Subsystem : Subsystem  Priority=11
  Subsystem1 : Subsystem  Priority=12
  Subsystem2 : Subsystem  Priority=13
  Subsystem3 : Subsystem  Priority=14
  Subsystem4 : Subsystem  Priority=11
  state_out : Outport
  wires:
  Subsystem3/1(state_out) -> state_out/1

== system compare_filters/no_LUT/hall_filter/First trigger initialization ==
  note: no need to shift because the hall signal here is already late by 1
  raw_hall : Inport
  Trigger : TriggerPort  VariantControl=(inherit)  PortDimensions=1
  Constant : Constant  Value=0
  Data Store Write3 : DataStoreWrite  DataStoreName=state_out  IndexOptions=Index vector (dialog)  Indices=1  OutputSizes=1
  MATLAB Function : MATLAB Function  TreatAsAtomicUnit=on
  Sum : Sum  Inputs=|+-
  wires:
  raw_hall/1 -> MATLAB Function/1(num)
  MATLAB Function/1(interval) -> Sum/1
  Sum/1 -> Data Store Write3/1
  Constant/1 -> Sum/2

== system compare_filters/no_LUT/hall_filter/calibration_routine ==
  note: $calculate ~\omega$
  note: $calculate ~\Delta\phi$
  note: $update ~LUT ~ table$
  function : TriggerPort  VariantControl=(inherit)
  Subsystem : Subsystem  Priority=11
  Subsystem1 : Subsystem  Priority=12
  Subsystem2 : Subsystem  Priority=13

== system compare_filters/no_LUT/hall_filter/hardware_ISR_routine ==
  note: partially resolved edge case: when hardware ISR and software ISR coincide
  note: 2. toggle timer reset
  note: 3. calculate tau's
  note: 4. calculate and register tau values into queue
  note: 1. save current time
  timer : Inport
  software_ISR_enable : Inport  Port=2
  omega_e : Inport  Port=3
  Trigger : TriggerPort  VariantControl=(inherit)  PortDimensions=1
  Atomic Subsystem : Subsystem  Priority=5  TreatAsAtomicUnit=on
  Bias : Bias  Bias=1  SaturateOnIntegerOverflow=off
  Constant : Constant  Value=use_LUT
  Constant7 : Constant  Value=phi_corr_LUT_param
  Data Store Memory : DataStoreMemory  DataStoreName=t_now  WriteAfterWriteMsg=warning  ShowAdditionalParam=off
  Data Store Memory1 : DataStoreMemory  DataStoreName=tau_corr_out  WriteAfterWriteMsg=warning  ShowAdditionalParam=off
  Data Store Read : DataStoreRead  DataStoreName=t_now  IndexOptions=Index vector (dialog)  Indices=1  OutputSizes=1
  Data Store Read1 : DataStoreRead  DataStoreName=tau_corr_now  IndexOptions=Index vector (dialog)  Indices=1  OutputSizes=1
  Data Store Read2 : DataStoreRead  DataStoreName=tau_corr_next  IndexOptions=Index vector (dialog)  Indices=1  OutputSizes=1
  Data Store Read3 : DataStoreRead  DataStoreName=tau_corr_out  IndexOptions=Index vector (dialog)  Indices=1  OutputSizes=1
  Data Store Read5 : DataStoreRead  DataStoreName=state_out  IndexOptions=Index vector (dialog)  Indices=1  OutputSizes=1
  Data Store Read6 : DataStoreRead  DataStoreName=state_out  IndexOptions=Index vector (dialog)  Indices=1  OutputSizes=1
  Data Store Write : DataStoreWrite  DataStoreName=tau_corr_out  IndexOptions=Index vector (dialog)  Indices=1  OutputSizes=1
  Divide : Product  Inputs=*/
  MATLAB Function : MATLAB Function  Priority=4  TreatAsAtomicUnit=on
  MATLAB Function1 : MATLAB Function  TreatAsAtomicUnit=on
  Scope : Scope
      settings: ActiveDisplayYMinimum=-0.027793962383284257  ActiveDisplayYMaximum=0.030008936086375265  DataLoggingVariableName=ScopeData4
  Selector : Selector  InputPortWidth=6  IndexOptions=Index vector (port)  Indices=[1 3]  OutputSizes=1
  Selector1 : Selector  InputPortWidth=6  IndexOptions=Index vector (port)  Indices=[1 3]  OutputSizes=1
  Subsystem : Subsystem  Priority=2  Commented=on
  Subsystem1 : Subsystem  Priority=3
  Subsystem2 : Subsystem  Priority=1
  Subsystem3 : Subsystem  Priority=5  Commented=on
  Unit Delay : UnitDelay  SampleTime=-1  HasFrameUpgradeWarning=on
  wires:
  Data Store Read/1 -> MATLAB Function/1(timer), Subsystem1/1(In1)
  Data Store Read1/1 -> MATLAB Function/3(tau_now)  "tau_corr_now"
  timer/1 -> Subsystem2/1(timer)
  Subsystem1/1(tau_vec) -> MATLAB Function/2(tau_vec)
  MATLAB Function/1(tau_now_out) -> Atomic Subsystem/1(tau_now_write)  "tau_now_write"
  MATLAB Function/2(tau_next_out) -> Atomic Subsystem/2(tau_next_write)  "tau_next_write"
  software_ISR_enable/1 -> Atomic Subsystem/Enable
  MATLAB Function/3(update_now) -> Atomic Subsystem/3(update_now)
  MATLAB Function/4(update_next) -> Atomic Subsystem/4(update_next)
  MATLAB Function/5(tau_corr_out) -> Data Store Write/1
  Data Store Read3/1 -> Scope/1  "tau_corr_out"
  Data Store Read2/1 -> MATLAB Function/4(tau_next)
  Constant/1 -> MATLAB Function/6(use_LUT)
  Constant7/1 -> Selector1/1, Divide/1
  Divide/1 -> MATLAB Function1/1(tau_LUT_input), Selector/1, MATLAB Function/5(tau_LUT_input)
  omega_e/1 -> Divide/2
  Bias/1 -> Selector1/2, Selector/2
  Selector/1 -> ?  "tau_corr_LUT"
  Data Store Read5/1 -> MATLAB Function/7(state_out)
  Selector1/1 -> ?  "phi_corr_test"
  Data Store Read6/1 -> Bias/1
  MATLAB Function1/1(tau_corr_LUT_test) -> ?  "tau_corr_LUT_algo"

== system compare_filters/no_LUT/hall_filter/software_ISR_routine ==
  note: turn off initialization flag
      | (only meaningful after initialization)
  note: advance switching state
  note: $\tau_\text{corr, next} -> \tau_\text{corr, now}$
  note: Update $\tau_\text{corr, next}$
  note: transfert state_out to output
  function : TriggerPort  VariantControl=(inherit)
  Subsystem : Subsystem  Priority=11
  Subsystem1 : Subsystem  Priority=12
  Subsystem2 : Subsystem  Priority=13
  Subsystem3 : Subsystem  Priority=14
  Subsystem4 : Subsystem  Priority=11
  state_out : Outport
  wires:
  Subsystem3/1(state_out) -> state_out/1

== system compare_filters/3_phase/hall_filter/calibration_routine/Subsystem ==
  Constant : Constant  Value=pi/3
  Data Store Read : DataStoreRead  DataStoreName=tau_corr_now  IndexOptions=Index vector (dialog)  Indices=1  OutputSizes=1
  Data Store Write : DataStoreWrite  DataStoreName=omega_now  IndexOptions=Index vector (dialog)  Indices=1  OutputSizes=1
  Divide : Product  Inputs=*/
  wires:
  Data Store Read/1 -> Divide/2
  Constant/1 -> Divide/1
  Divide/1 -> Data Store Write/1

== system compare_filters/3_phase/hall_filter/calibration_routine/Subsystem1 ==
  Data Store Read : DataStoreRead  DataStoreName=tau_corr_now  IndexOptions=Index vector (dialog)  Indices=1  OutputSizes=1
  Data Store Read1 : DataStoreRead  DataStoreName=omega_now  IndexOptions=Index vector (dialog)  Indices=1  OutputSizes=1
  Data Store Write : DataStoreWrite  DataStoreName=del_phi  IndexOptions=Index vector (dialog)  Indices=1  OutputSizes=1
  Product : Product
  wires:
  Data Store Read/1 -> Product/1
  Data Store Read1/1 -> Product/2
  Product/1 -> Data Store Write/1

== system compare_filters/3_phase/hall_filter/calibration_routine/Subsystem2 ==
  Constant : Constant  Value=6
  Constant1 : Constant  Value=0.02
  Constant2 : Constant  Value=4e-4
  Constant3 : Constant  Value=50
  Data Store Read1 : DataStoreRead  DataStoreName=state_out  IndexOptions=Index vector (dialog)  Indices=1  OutputSizes=1
  Data Store Read2 : DataStoreRead  DataStoreName=del_phi  IndexOptions=Index vector (dialog)  Indices=1  OutputSizes=1
  Data Store Read3 : DataStoreRead  DataStoreName=LUT_phi  IndexOptions=Index vector (dialog)  Indices=1  OutputSizes=1
  Data Store Read4 : DataStoreRead  DataStoreName=LUT_var  IndexOptions=Index vector (dialog)  Indices=1  OutputSizes=1
  Data Store Read5 : DataStoreRead  DataStoreName=LUT_count  IndexOptions=Index vector (dialog)  Indices=1  OutputSizes=1
  Data Store Read6 : DataStoreRead  DataStoreName=LUT_valid  IndexOptions=Index vector (dialog)  Indices=1  OutputSizes=1
  Data Store Read7 : DataStoreRead  DataStoreName=cal_done  IndexOptions=Index vector (dialog)  Indices=1  OutputSizes=1
  Data Store Write : DataStoreWrite  DataStoreName=LUT_phi  IndexOptions=Index vector (dialog)  Indices=1  OutputSizes=1
  Data Store Write1 : DataStoreWrite  DataStoreName=LUT_var  IndexOptions=Index vector (dialog)  Indices=1  OutputSizes=1
  Data Store Write2 : DataStoreWrite  DataStoreName=LUT_count  IndexOptions=Index vector (dialog)  Indices=1  OutputSizes=1
  Data Store Write3 : DataStoreWrite  DataStoreName=LUT_valid  IndexOptions=Index vector (dialog)  Indices=1  OutputSizes=1
  Data Store Write4 : DataStoreWrite  DataStoreName=cal_done  IndexOptions=Index vector (dialog)  Indices=1  OutputSizes=1
  MATLAB Function : MATLAB Function  TreatAsAtomicUnit=on
  wires:
  Data Store Read1/1 -> MATLAB Function/1(k)
  Data Store Read2/1 -> MATLAB Function/2(dphi)
  Data Store Read3/1 -> MATLAB Function/3(phi)
  Data Store Read4/1 -> MATLAB Function/4(varv)
  Data Store Read5/1 -> MATLAB Function/5(cnt)
  Data Store Read6/1 -> MATLAB Function/6(valid)
  Data Store Read7/1 -> MATLAB Function/7(done)
  Constant/1 -> MATLAB Function/8(Nsteady)
  Constant1/1 -> MATLAB Function/9(deadband_rad)
  Constant2/1 -> MATLAB Function/10(var_max)
  Constant3/1 -> MATLAB Function/11(omega_min)
  MATLAB Function/1(phi_n) -> Data Store Write/1
  MATLAB Function/2(varv_n) -> Data Store Write1/1
  MATLAB Function/3(cnt_n) -> Data Store Write2/1
  MATLAB Function/4(valid_n) -> Data Store Write3/1
  MATLAB Function/5(done_n) -> Data Store Write4/1

== system compare_filters/3_phase/hall_filter/hardware_ISR_routine/Atomic Subsystem ==
  tau_now_write : Inport
  tau_next_write : Inport  Port=2
  update_now : Inport  Port=3
  update_next : Inport  Port=4
  software_ISR_enable : EnablePort
  Subsystem : Subsystem
  Subsystem1 : Subsystem
  wires:
  tau_next_write/1 -> Subsystem1/1(tau_next_write)
  update_now/1 -> Subsystem/Enable
  update_next/1 -> Subsystem1/Enable
  tau_now_write/1 -> Subsystem/1(tau_now_write)

== system compare_filters/3_phase/hall_filter/hardware_ISR_routine/Subsystem ==
  Constant : Constant
  Data Store Read : DataStoreRead  DataStoreName=reset_toggle  IndexOptions=Index vector (dialog)  Indices=1  OutputSizes=1
  Data Store Read1 : DataStoreRead  DataStoreName=time_base  IndexOptions=Index vector (dialog)  Indices=1  OutputSizes=1
  Data Store Read2 : DataStoreRead  DataStoreName=t_now  IndexOptions=Index vector (dialog)  Indices=1  OutputSizes=1
  Data Store Write : DataStoreWrite  DataStoreName=reset_toggle  IndexOptions=Index vector (dialog)  Indices=1  OutputSizes=1
  Data Store Write1 : DataStoreWrite  DataStoreName=time_base  IndexOptions=Index vector (dialog)  Indices=1  OutputSizes=1
  Sum : Sum  Inputs=|-+
  Sum1 : Sum  Inputs=|++
  wires:
  Sum/1 -> Data Store Write/1  "reset_val"
  Data Store Read/1 -> Sum/1
  Constant/1 -> Sum/2
  Data Store Read1/1 -> Sum1/1
  Sum1/1 -> Data Store Write1/1
  Data Store Read2/1 -> Sum1/2
